simulink model "BLDCTest"  (R2014b)
settings: Solver=ode45  StartTime=0.0  StopTime=.3  MaxStep=.0001  RelTol=1e-3
libraries: simulink x1

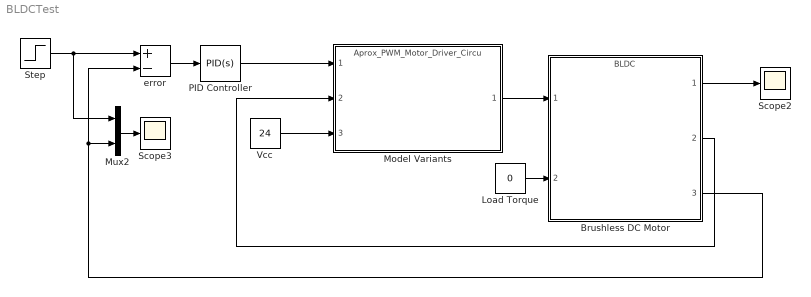
== system BLDCTest ==
  Brushless DC Motor : ModelReference  ModelNameDialog=BLDC  SimulationMode=Normal  ModelReferenceVersion=1.178  CopyOfModelName=BLDC  DefaultDataLogging=on
  Load Torque : Constant  Value=0
  Model Variants : ModelReference  ModelNameDialog=Aprox_PWM_Motor_Driver_Circu.slx  SimulationMode=Normal  Variant=on  ModelReferenceVersion=1.196  CopyOfModelName=Aprox_PWM_Motor_Driver_Circu.slx  DefaultDataLogging=on
  Mux2 : Mux  Inputs=2
  PID Controller : simulink/Continuous/PID Controller  Controller=PID  TimeDomain=Continuous-time  SampleTime=-1  IntegratorMethod=Forward Euler  FilterMethod=Forward Euler  Form=Parallel  P=50  I=10  D=0  N=100  InitialConditionSource=internal  InitialConditionForIntegrator=0  InitialConditionForFilter=0  ExternalReset=none  LimitOutput=off  UpperSaturationLimit=inf  LowerSaturationLimit=-inf  LinearizeAsGain=on  AntiWindupMode=none  Kb=1  TrackingMode=off  Kt=1  PParamMin=[]  PParamMax=[]  IParamMin=[]  IParamMax=[]  DParamMin=[]  DParamMax=[]  NParamMin=[]  NParamMax=[]  KbParamMin=[]  KbParamMax=[]  KtParamMin=[]  KtParamMax=[]  POutMin=[]  POutMax=[]  IOutMin=[]  IOutMax=[]  DOutMin=[]  DOutMax=[]  NOutMin=[]  NOutMax=[]  KbOutMin=[]  KbOutMax=[]  KtOutMin=[]  KtOutMax=[]  IntegratorOutMin=[]  IntegratorOutMax=[]  FilterOutMin=[]  FilterOutMax=[]  SumOutMin=[]  SumOutMax=[]  SumI1OutMin=[]  SumI1OutMax=[]  SumI2OutMin=[]  SumI2OutMax=[]  SumI3OutMin=[]  SumI3OutMax=[]  SumDOutMin=[]  SumDOutMax=[]  SaturationOutMin=[]  SaturationOutMax=[]  IntegratorContinuousStateAttributes=''  IntegratorStateMustResolveToSignalObject=off  IntegratorRTWStateStorageClass=Auto  FilterContinuousStateAttributes=''  FilterStateMustResolveToSignalObject=off  FilterRTWStateStorageClass=Auto  DifferentiatorICPrevScaledInput=0  DifferentiatorOutMin=[]  DifferentiatorOutMax=[]  UseFilter=on
  Scope2 : Scope
  Scope3 : Scope
  Step : Step  Time=.1  After=2*pi  SampleTime=0
  Vcc : Constant  Value=24
  error : Sum  Inputs=+-
  wires:
  error/1 -> PID Controller/1
  Mux2/1 -> Scope3/1
  Step/1 -> Mux2/1, error/1
  Brushless DC Motor/3 -> error/2, Mux2/2
  Load Torque/1 -> Brushless DC Motor/2
  Brushless DC Motor/1 -> Scope2/1
  PID Controller/1 -> Model Variants/1
  Vcc/1 -> Model Variants/3
  Model Variants/1 -> Brushless DC Motor/1
  Brushless DC Motor/2 -> Model Variants/2
